simulink model "O1"  (Simulink 8.8)
settings: Solver=ode45  StartTime=0.0  StopTime=10.0  RelTol=1e-3  EnableMultiTasking=on
settings Model: Creator=Bonner  LastModifiedBy=Bonner
settings DataIOCC: LimitDataPoints=off  SignalLoggingSaveFormat=Dataset  InspectSignalLogs=on
settings OptimizationCC: LifeSpan=auto
settings DebuggingCC: UnderspecifiedInitializationDetection=Simplified  MergeDetectMultiDrivingBlocksExec=error  FcnCallInpInsideContextMsg=error  StateNameClashWarn=none  SFUnexpectedBacktrackingDiag=error  SFNoUnconditionalDefaultTransitionDiag=error
settings HardwareCC: ProdBitPerPointer=64  ProdBitPerSizeT=64  ProdBitPerPtrDiffT=64  ProdLargestAtomicFloat=Float  ProdIntDivRoundTo=Zero  ProdEndianess=LittleEndian  ProdWordSize=64  ProdHWDeviceType=Intel->x86-64 (Windows64)
settings ModelReferenceCC: PropagateSignalLabelsOutOfModel=on
settings GRTTargetCC: TargetLangStandard=C99 (ISO)  GeneratePreprocessorConditionals=Use local settings  CombineOutputUpdateFcns=on  GRTInterface=off
settings ConfigComp: CovSFcnEnable=off

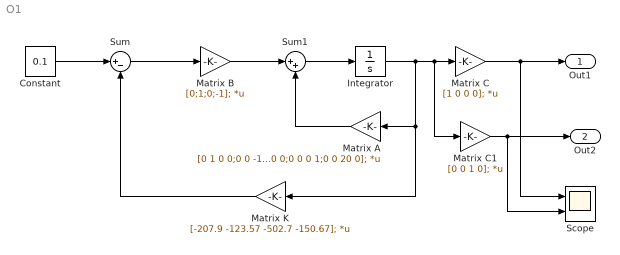
== system O1 ==
  Constant : Constant  Value=0.1
  Integrator : Integrator  InitialCondition=[0 0 0.1 0]
  Matrix A : Gain  Gain=[0 1 0 0;0 0 -10 0;0 0 0 1;0 0 20 0];  Multiplication=Matrix(K*u)
  Matrix B : Gain  Gain=[0;1;0;-1];  Multiplication=Matrix(K*u)
  Matrix C : Gain  Gain=[1 0 0 0];  Multiplication=Matrix(K*u)
  Matrix C1 : Gain  Gain=[0 0 1 0];  Multiplication=Matrix(K*u)
  Matrix K : Gain  Gain=[-207.9 -123.57 -502.7 -150.67];  Multiplication=Matrix(K*u)
  Scope : Scope  NumInputPorts=2
  Sum : Sum  Inputs=|+-
  Sum1 : Sum  Inputs=|++
  Out1 : Outport
  Out2 : Outport  Port=2
  wires:
  Sum/1 -> Matrix B/1
  Matrix B/1 -> Sum1/1
  Sum1/1 -> Integrator/1
  Integrator/1 -> Matrix K/1, Matrix A/1, Matrix C1/1, Matrix C/1
  Matrix C/1 -> Scope/1, Out1/1
  Matrix A/1 -> Sum1/2
  Matrix K/1 -> Sum/2
  Constant/1 -> Sum/1
  Matrix C1/1 -> Out2/1, Scope/2
